simulink model "SMC_stateflow_model"  (R2022a)
settings: Solver=VariableStepAuto  StartTime=0.0  StopTime=20  FixedStep=0.1  MaxStep=1e-3  RelTol=1e-3  EnableMultiTasking=on
InitFcn:
  | clear
  | clc
  | %% dati
  | w0 = 5.278;
  | alfa1 = w0^2;
  | alfa3 = -1.402*w0^2;
  | alfa5 = 0.271*w0^2;
  | mu1 = 0.086;
  | mu3 = 0.1080;
  | %% parametri SMC
  | mu = 20;
  | P = [1 3]';
  | x0 = [-1.2 -0.18]';
  | xd = [0 0]';
  | Ad = 5; %ampiezza disturbo
  | fd = 2; %frequenza disturbo
  | epsilon = 0.1; %boundary layer
settings Model: Creator=user  LastModifiedBy=user
settings SolverCC: ZeroCrossAlgorithm=Adaptive  AlgebraicLoopSolver=TrustRegion  AutoInsertRateTranBlk=on
settings DataIOCC: LimitDataPoints=on
settings OptimizationCC: LifeSpan=inf
settings DebuggingCC: IgnoredZcDiagnostic=none  UnconnectedInputMsg=warning  UnconnectedOutputMsg=warning  UnconnectedLineMsg=warning  AllowSymbolicDim=off  SFUnexpectedBacktrackingDiag=warning  SFNoUnconditionalDefaultTransitionDiag=warning  SFExecutionAtInitializationDiag=none  ArithmeticOperatorsInVariantConditions=warning
settings SFSimCC: SimUseLocalCustomCode=off  CustomCodeUndefinedFunction=UseInterfaceOnly
settings RTWCC: RTWUseLocalCustomCode=off  DLArmComputeVersion=19.05
settings CodeAppCC: StateflowObjectComments=on
settings GRTTargetCC: TargetLangStandard=C89/C90 (ANSI)
settings ConfigComp: CovMetricSettings=dw  CovSaveCumulativeToWorkspaceVar=on  CovSaveSingleToWorkspaceVar=on  CovExternalEMLEnable=off  CovSFcnEnable=off

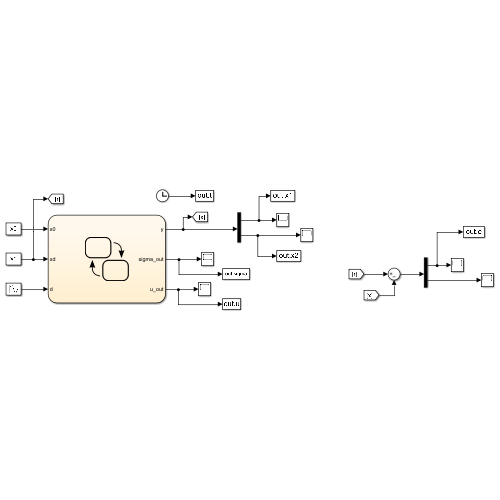
[thumbnail: Simulink's stored preview of the top-level diagram]
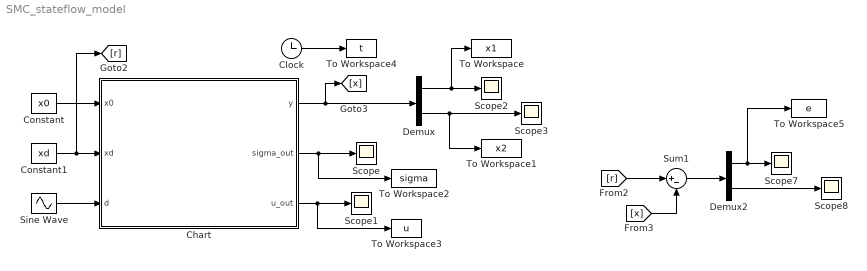
== system SMC_stateflow_model ==
  Chart : Stateflow chart  TreatAsAtomicUnit=on
  Clock : Clock
  Constant : Constant  Value=x0
  Constant1 : Constant  Value=xd
  Demux : Demux  Outputs=2
  Demux2 : Demux  Outputs=2
  Scope{,1..3,7..8} (6 alike) : Scope
  Sine Wave : Sin  Amplitude=Ad  SampleTime=0
  Sum1 : Sum  Inputs=|+-
  To Workspace : ToWorkspace  VariableName=x1  SampleTime=-1
      settings: Save2DSignal=2-D array (concatenate along first dimension)
  To Workspace1 : ToWorkspace  VariableName=x2  SampleTime=-1
      settings: Save2DSignal=2-D array (concatenate along first dimension)
  To Workspace2 : ToWorkspace  VariableName=sigma  SampleTime=-1
      settings: Save2DSignal=2-D array (concatenate along first dimension)
  To Workspace3 : ToWorkspace  VariableName=u  SampleTime=-1
      settings: Save2DSignal=2-D array (concatenate along first dimension)
  To Workspace4 : ToWorkspace  VariableName=t  SampleTime=-1
      settings: Save2DSignal=2-D array (concatenate along first dimension)
  To Workspace5 : ToWorkspace  VariableName=e  SampleTime=-1
      settings: Save2DSignal=2-D array (concatenate along first dimension)
  wires:
  Constant/1 -> Chart/1(x0)
  Constant1/1 -> [r], Chart/2(xd)
  Sine Wave/1 -> Chart/3(d)
  Chart/2(sigma_out) -> To Workspace2/1, Scope/1
  Chart/1(y) -> [x], Demux/1
  Demux/2 -> To Workspace1/1, Scope3/1
  Demux/1 -> Scope2/1, To Workspace/1
  Chart/3(u_out) -> To Workspace3/1, Scope1/1
  Clock/1 -> To Workspace4/1
  [r] -> Sum1/1
  [x] -> Sum1/2
  Sum1/1 -> Demux2/1
  Demux2/1 -> To Workspace5/1, Scope7/1
  Demux2/2 -> Scope8/1

== stateflow chart SMC_stateflow_model/Chart ==
  settings: updateMethod=CONTINUOUS
  state roll_plus_mode
    during:
    x_dot = Fp;
    y = x;
    sigma_out = sigma;
    u_out = u_eq+u_sw_p;
  state roll_minus_mode
    during:
    x_dot = Fm;
    y = x;
    sigma_out = sigma;
    u_out = u_eq+u_sw_m;
  state roll_init
    en:
    x=x0;
    y = x;
    sigma_out = sigma;
    u_out = 0;
  state roll_sliding_mode
    during:
    x_dot = Fs;
    y = x;
    sigma_out = sigma;
    u_out = u_eq;
  roll_init -> roll_minus_mode [order 2] : [sigma < 0]
  (default) -> roll_init
  roll_plus_mode -> roll_minus_mode [order 1] : [sigma<=0 && L_Fp_sigma*L_Fm_sigma>=0]
  roll_init -> roll_plus_mode [order 1] : [sigma > 0]
  roll_minus_mode -> roll_plus_mode [order 1] : [sigma>=0 && L_Fp_sigma*L_Fm_sigma>=0]
  roll_init -> roll_sliding_mode [order 3] : [sigma == 0]
  roll_sliding_mode -> roll_plus_mode [order 1] : [L_Fp_sigma >0 && L_Fm_sigma >=0]
  roll_plus_mode -> roll_sliding_mode [order 2] : [sigma<=0 && L_Fm_sigma>=0 && L_Fp_sigma<=0]
  roll_minus_mode -> roll_sliding_mode [order 2] : [sigma>=0 && L_Fm_sigma>=0 && L_Fp_sigma<=0]
  roll_sliding_mode -> roll_minus_mode [order 2] : [L_Fp_sigma<=0 && L_Fm_sigma<0]
  data: u_eq_val function_output; u_sw_p_val function_output; u_sw_m_val function_output; sigma_val function_output; Fp_val function_output; Fm_val function_output; Fs_val function_output; L_Fp_sigma_val function_output; L_Fm_sigma_val function_output; x local; y output; sigma_out output; u_out output; x0 input; xd input; d input; mu parameter; mu1 parameter; mu3 parameter; alfa1 parameter; alfa3 parameter; alfa5 parameter; P parameter
  data x settings: updateMethod=SF_CONTINUOUS_TIME_DATA
  function u_eq_val = u_eq:
    | function u_eq_val = u_eq
    | 
    | u_eq_val = -(P(1)/P(2))*x(2) + 2*mu1*x(2) + mu3*x(2)^3 + alfa1*x(1) + alfa3*x(1)^3 + alfa5*x(1)^5;
    | 
    | end
  function u_sw_p_val = u_sw_p:
    | function u_sw_p_val = u_sw_p
    | 
    | u_sw_p_val = -mu/P(2);
    | 
    | end
  function u_sw_m_val = u_sw_m:
    | function u_sw_m_val = u_sw_m
    | 
    | u_sw_m_val = mu/P(2);
    | 
    | end
  function sigma_val = sigma:
    | function sigma_val = sigma
    | 
    | sigma_val = P' * (x-xd);
    | 
    | end
  function Fp_val = Fp:
    | function Fp_val = Fp
    | 
    | u = u_eq + u_sw_p;
    | Fp_val = [x(2);... 
    |           -2*mu1*x(2) - mu3*x(2)^3 - alfa1*x(1) - alfa3*x(1)^3 - alfa5*x(1)^5 + d + u];
    | 
    | end
  function Fm_val = Fm:
    | function Fm_val = Fm
    | 
    | u = u_eq + u_sw_m;
    | Fm_val = [x(2);... 
    |           -2*mu1*x(2) - mu3*x(2)^3 - alfa1*x(1) - alfa3*x(1)^3 - alfa5*x(1)^5 + d + u];
    | 
    | end
  function Fs_val = Fs:
    | function Fs_val = Fs
    | 
    | Fs_val = [-(P(1)/P(2))*x(1); -(P(1)/P(2))*x(2)];
    | 
    | end
  function L_Fp_sigma_val = L_Fp_sigma:
    | function L_Fp_sigma_val = L_Fp_sigma
    | 
    | L_Fp_sigma_val = P' * Fp;
    | 
    | end
  function L_Fm_sigma_val = L_Fm_sigma:
    | function L_Fm_sigma_val = L_Fm_sigma
    | 
    | L_Fm_sigma_val = P' * Fm;
    | 
    | end
